simulink library "simInfo_ld_common_v0"  (R2016a)
settings: Solver=ode45  StartTime=0.0  StopTime=10.0  RelTol=1e-3
libraries: simulink x1
settings Model: Creator=uwlelke  LastModifiedBy=UWLELKE
settings DataIOCC: LimitDataPoints=on  SaveFormat=Array
settings DebuggingCC: SolverPrmCheckMsg=warning
settings HardwareCC: ProdBitPerPointer=32  ProdLargestAtomicFloat=None  ProdIntDivRoundTo=Undefined  ProdEndianess=Unspecified  ProdWordSize=32  ProdHWDeviceType=32-bit Generic
settings ModelReferenceCC: PropagateSignalLabelsOutOfModel=off
settings ConfigComp: CovModelRefEnable=Off  CovSFcnEnable=off

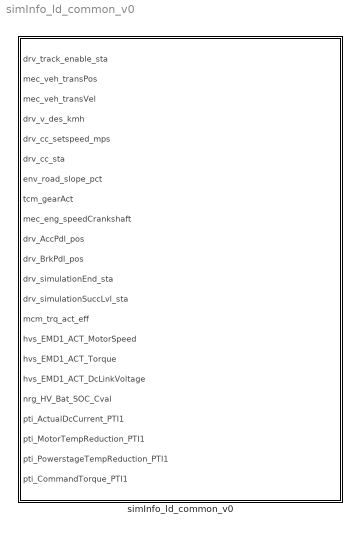
== system simInfo_ld_common_v0 ==
  simInfo_ld_common_v0 : Subsystem  VariantControl=voSimInfo_SIMINFO

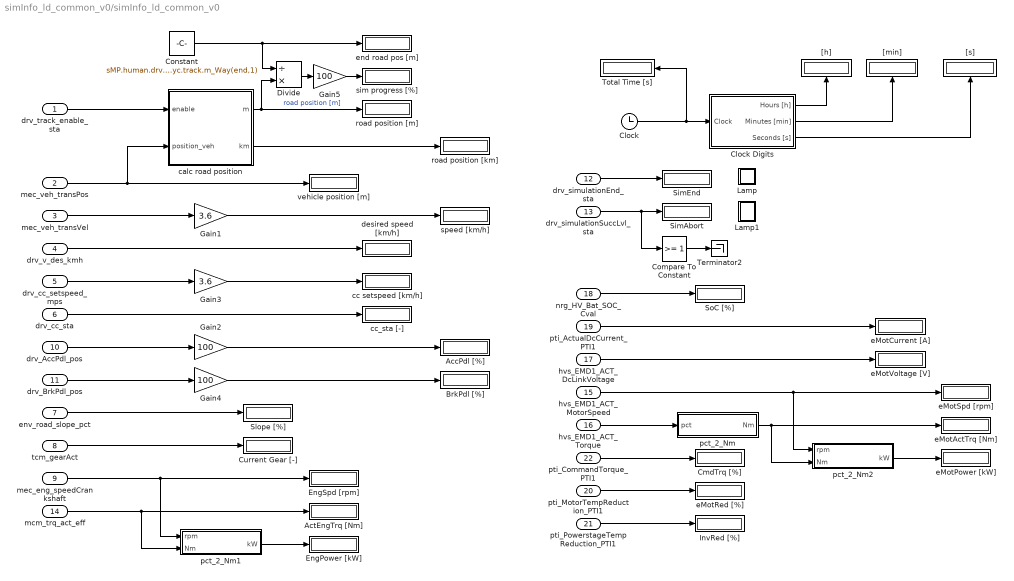
== system simInfo_ld_common_v0/simInfo_ld_common_v0 ==
  drv_track_enable_sta : Inport
  mec_veh_transPos : Inport  Port=2
  mec_veh_transVel : Inport  Port=3
  drv_v_des_kmh : Inport  Port=4
  drv_cc_setspeed_mps : Inport  Port=5
  drv_cc_sta : Inport  Port=6
  env_road_slope_pct : Inport  Port=7
  tcm_gearAct : Inport  Port=8
  mec_eng_speedCrankshaft : Inport  Port=9
  drv_AccPdl_pos : Inport  Port=10
  drv_BrkPdl_pos : Inport  Port=11
  drv_simulationEnd_sta : Inport  Port=12
  drv_simulationSuccLvl_sta : Inport  Port=13
  mcm_trq_act_eff : Inport  Port=14
  hvs_EMD1_ACT_MotorSpeed : Inport  Port=15
  hvs_EMD1_ACT_Torque : Inport  Port=16
  hvs_EMD1_ACT_DcLinkVoltage : Inport  Port=17
  nrg_HV_Bat_SOC_Cval : Inport  Port=18
  pti_ActualDcCurrent_PTI1 : Inport  Port=19
  pti_MotorTempReduction_PTI1 : Inport  Port=20
  pti_PowerstageTempReduction_PTI1 : Inport  Port=21
  pti_CommandTorque_PTI1 : Inport  Port=22
  AccPdl [%] : Display
      settings: Format=bank
  ActEngTrq [Nm] : Display
      settings: Format=bank
  BrkPdl [%] : Display
      settings: Format=bank
  Clock : Clock
  Clock Digits : Subsystem
  CmdTrq [%] : Display
      settings: Format=bank
  Compare To Constant : simulink/Logic and Bit Operations/Compare To Constant  relop=>=  const=1  OutDataTypeStr=boolean
  Constant : Constant  Value=sMP.human.drv.cyc.track.m_Way(end,1)
      settings: AttributesFormatString=%<Value>
  Current Gear [-] : Display
      settings: Decimation=2
  Divide : Product  Inputs=/*
  EngPower [kW] : Display
      settings: Format=bank
  EngSpd [rpm] : Display
      settings: Format=bank
  Gain1 : Gain  Gain=3.6
  Gain2 : Gain  Gain=100
  Gain3 : Gain  Gain=3.6
  Gain4 : Gain  Gain=100
  Gain5 : Gain  Gain=100
  InvRed [%] : Display
      settings: Format=bank
  Lamp : Subsystem  Description=SimEnd  DialogController=hmiCreateDDGDialog  IsWebBlock=on  mask(MWDashboardBlock){webBlockId=dbaadf46-52fa-43c2-9fa4-8f0c76259098, webBlockType=lamp, ShowInLibBrowser=on, ShowInitialText=on, HMISrcModelName=DIVeMB_Model}
      mask prompts: webBlockType "WebBlock Type"; HMISrcModelName "Source Model"
      settings: AttributesFormatString=%<Description>
      mask Help: helpview([docroot '/mapfiles/simulink.map'], 'hmi_lamp')
      mask Display:
      | if strcmp(get_param(bdroot(gcb),'BlockDiagramType'), 'library')
      |     image([(matlabroot) '/toolbox/simulink/hmi/icons/Lamp.png']);
      | end
  Lamp1 : Subsystem  Description=SimAbort  DialogController=hmiCreateDDGDialog  IsWebBlock=on  mask(MWDashboardBlock){webBlockId=598b827d-4754-44fa-abcb-4d247324de2c, webBlockType=lamp, ShowInLibBrowser=on, ShowInitialText=on, HMISrcModelName=DIVeMB_Model}
      mask prompts: webBlockType "WebBlock Type"; HMISrcModelName "Source Model"
      settings: AttributesFormatString=%<Description>
      mask Help: helpview([docroot '/mapfiles/simulink.map'], 'hmi_lamp')
      mask Display:
      | if strcmp(get_param(bdroot(gcb),'BlockDiagramType'), 'library')
      |     image([(matlabroot) '/toolbox/simulink/hmi/icons/Lamp.png']);
      | end
  SimAbort : Display
  SimEnd : Display
  Slope [%] : Display
      settings: Format=bank
  SoC [%] : Display
      settings: Format=bank
  Terminator2 : Terminator
  Total Time [s] : Display
      settings: Format=bank
  "[h]" : Display
  "[min]" : Display
  "[s]" : Display
      settings: Format=bank
  calc road position : Subsystem
  cc setspeed [km/h] : Display
      settings: Format=bank
  cc_sta [-] : Display
      settings: Format=bank
  desired speed [km/h] : Display
      settings: Format=bank
  eMotActTrq [Nm] : Display
      settings: Format=bank
  eMotCurrent [A] : Display
      settings: Format=bank
  eMotPower [kW] : Display
      settings: Format=bank
  eMotRed [%] : Display
      settings: Format=bank
  eMotSpd [rpm] : Display
      settings: Format=bank
  eMotVoltage [V] : Display
      settings: Format=bank
  end road pos [m] : Display
      settings: Format=bank
  pct_2_Nm : Subsystem
  pct_2_Nm1 : Subsystem
  pct_2_Nm2 : Subsystem
  road position [km] : Display
      settings: Format=bank
  road position [m] : Display
      settings: Format=bank
  sim progress [%] : Display
      settings: Format=bank
  speed [km/h] : Display
      settings: Format=bank
  vehicle position [m] : Display
      settings: Format=bank
  wires:
  pti_CommandTorque_PTI1/1 -> CmdTrq [%]/1
  nrg_HV_Bat_SOC_Cval/1 -> SoC [%]/1
  hvs_EMD1_ACT_DcLinkVoltage/1 -> eMotVoltage [V]/1
  pct_2_Nm2/1(kW) -> eMotPower [kW]/1
  pct_2_Nm1/1(kW) -> EngPower [kW]/1
  pct_2_Nm/1(Nm) -> eMotActTrq [Nm]/1, pct_2_Nm2/2(Nm)
  hvs_EMD1_ACT_Torque/1 -> pct_2_Nm/1(pct)
  hvs_EMD1_ACT_MotorSpeed/1 -> eMotSpd [rpm]/1, pct_2_Nm2/1(rpm)
  drv_cc_sta/1 -> cc_sta [-]/1
  Constant/1 -> Divide/1, end road pos [m]/1
  calc road position/1(m) -> Divide/2, road position [m]/1  "road position [m]"
  calc road position/2(km) -> road position [km]/1
  drv_track_enable_sta/1 -> calc road position/1(enable)
  Gain1/1 -> speed [km/h]/1
  Gain2/1 -> AccPdl [%]/1
  drv_BrkPdl_pos/1 -> Gain4/1
  drv_AccPdl_pos/1 -> Gain2/1
  drv_cc_setspeed_mps/1 -> Gain3/1
  drv_v_des_kmh/1 -> desired speed [km/h]/1
  Gain3/1 -> cc setspeed [km/h]/1
  drv_simulationSuccLvl_sta/1 -> Compare To Constant/1, SimAbort/1
  drv_simulationEnd_sta/1 -> SimEnd/1
  mcm_trq_act_eff/1 -> pct_2_Nm1/2(Nm), ActEngTrq [Nm]/1
  mec_eng_speedCrankshaft/1 -> pct_2_Nm1/1(rpm), EngSpd [rpm]/1
  env_road_slope_pct/1 -> Slope [%]/1
  tcm_gearAct/1 -> Current Gear [-]/1
  Clock Digits/1(Hours [h]) -> "[h]"/1
  Clock Digits/2(Minutes [min]) -> "[min]"/1
  Clock Digits/3(Seconds [s]) -> "[s]"/1
  Clock/1 -> Clock Digits/1(Clock), Total Time [s]/1
  mec_veh_transPos/1 -> calc road position/2(position_veh), vehicle position [m]/1
  mec_veh_transVel/1 -> Gain1/1
  pti_ActualDcCurrent_PTI1/1 -> eMotCurrent [A]/1
  pti_MotorTempReduction_PTI1/1 -> eMotRed [%]/1
  pti_PowerstageTempReduction_PTI1/1 -> InvRed [%]/1
  Divide/1 -> Gain5/1
  Gain5/1 -> sim progress [%]/1
  Compare To Constant/1 -> Terminator2/1
  Gain4/1 -> BrkPdl [%]/1

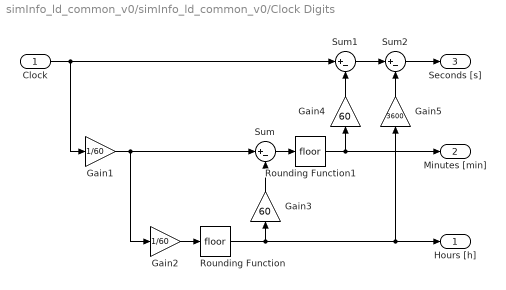
== system simInfo_ld_common_v0/simInfo_ld_common_v0/Clock Digits ==
  Clock : Inport
  Gain1 : Gain  Gain=1/60
  Gain2 : Gain  Gain=1/60
  Gain3 : Gain  Gain=60
  Gain4 : Gain  Gain=60
  Gain5 : Gain  Gain=3600
  Rounding Function : Rounding
  Rounding Function1 : Rounding
  Sum : Sum  Inputs=|+-
  Sum1 : Sum  Inputs=|+-
  Sum2 : Sum  Inputs=|+-
  Hours [h] : Outport
  Minutes [min] : Outport  Port=2
  Seconds [s] : Outport  Port=3
  wires:
  Gain1/1 -> Gain2/1, Sum/1
  Gain2/1 -> Rounding Function/1
  Rounding Function/1 -> Gain3/1, Hours [h]/1, Gain5/1
  Gain3/1 -> Sum/2
  Sum/1 -> Rounding Function1/1
  Rounding Function1/1 -> Gain4/1, Minutes [min]/1
  Gain4/1 -> Sum1/2
  Clock/1 -> Sum1/1, Gain1/1
  Sum1/1 -> Sum2/1
  Sum2/1 -> Seconds [s]/1
  Gain5/1 -> Sum2/2

== system simInfo_ld_common_v0/simInfo_ld_common_v0/Lamp ==

== system simInfo_ld_common_v0/simInfo_ld_common_v0/Lamp1 ==

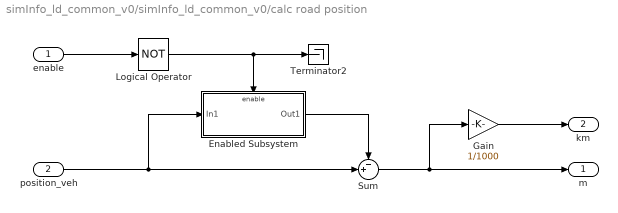
== system simInfo_ld_common_v0/simInfo_ld_common_v0/calc road position ==
  enable : Inport
  position_veh : Inport  Port=2
  Enabled Subsystem : Subsystem  TreatAsAtomicUnit=on
  Gain : Gain  Gain=1/1000
      settings: AttributesFormatString=%<Gain>
  Logical Operator : Logic  Operator=NOT  AllPortsSameDT=off  OutDataTypeStr=boolean
  Sum : Sum  Inputs=-+|
  Terminator2 : Terminator
  m : Outport
  km : Outport  Port=2
  wires:
  position_veh/1 -> Sum/2, Enabled Subsystem/1(In1)
  Sum/1 -> Gain/1, m/1
  Gain/1 -> km/1
  enable/1 -> Logical Operator/1
  Logical Operator/1 -> Terminator2/1, Enabled Subsystem/Enable
  Enabled Subsystem/1(Out1) -> Sum/1

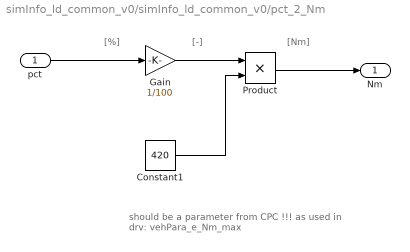
== system simInfo_ld_common_v0/simInfo_ld_common_v0/pct_2_Nm ==
  note: [-]
  note: [%]
  note: [Nm]
  note: should be a parameter from CPC !!!
      |
      | as used in drv: vehPara_e_Nm_max
  pct : Inport
  Constant1 : Constant  Value=420
      settings: AttributesFormatString=%<Value>
  Gain : Gain  Gain=1/100
      settings: AttributesFormatString=%<Gain>
  Product : Product
  Nm : Outport
  wires:
  pct/1 -> Gain/1
  Product/1 -> Nm/1
  Constant1/1 -> Product/2
  Gain/1 -> Product/1

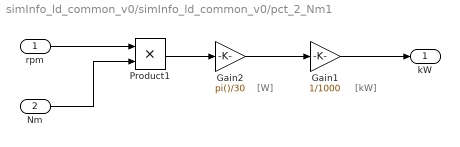
== system simInfo_ld_common_v0/simInfo_ld_common_v0/pct_2_Nm1 ==
  note: [W]
  note: [kW]
  rpm : Inport
  Nm : Inport  Port=2
  Gain1 : Gain  Gain=1/1000
      settings: AttributesFormatString=%<Gain>
  Gain2 : Gain  Gain=pi()/30
      settings: AttributesFormatString=%<Gain>
  Product1 : Product
  kW : Outport
  wires:
  Gain2/1 -> Gain1/1
  Product1/1 -> Gain2/1
  Nm/1 -> Product1/2
  Gain1/1 -> kW/1
  rpm/1 -> Product1/1

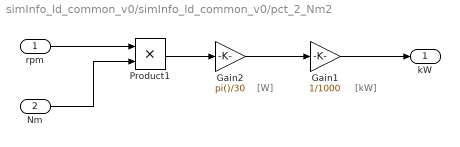
== system simInfo_ld_common_v0/simInfo_ld_common_v0/pct_2_Nm2 ==
  note: [kW]
  note: [W]
  rpm : Inport
  Nm : Inport  Port=2
  Gain1 : Gain  Gain=1/1000
      settings: AttributesFormatString=%<Gain>
  Gain2 : Gain  Gain=pi()/30
      settings: AttributesFormatString=%<Gain>
  Product1 : Product
  kW : Outport
  wires:
  rpm/1 -> Product1/1
  Gain1/1 -> kW/1
  Nm/1 -> Product1/2
  Product1/1 -> Gain2/1
  Gain2/1 -> Gain1/1

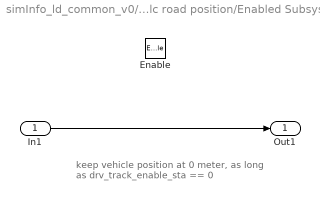
== system simInfo_ld_common_v0/simInfo_ld_common_v0/calc road position/Enabled Subsystem ==
  note: keep vehicle position at 0 meter,
      | as long as drv_track_enable_sta == 0
  In1 : Inport
  Enable : EnablePort
  Out1 : Outport
  wires:
  In1/1 -> Out1/1
